simulink model "Final_Model_Building_2_AirflowAdded"  (R2022a)
settings: Solver=ode1  StartTime=0.0  StopTime=24*3600  FixedStep=10  RelTol=1e-3
values from neighbouring files (symbols this model uses):
  Aux_Threshold = 52    [Setup_Code_EWASP_VC.m]
  buildingAge = 2005    [Setup_Code_EWASP_VC.m]
  ceilingHeight = 2.4    [Setup_Code_EWASP_VC.m]
  conductiveHconnectMatrix = [ ... (first row only)    [Setup_Code_EWASP_VC.m]
  cRoofGreen = 100000    [Setup_Code_EWASP_VC.m]
  Defrost_After_Time = 30    [Setup_Code_EWASP_VC.m]
  DHWDemandProfile = occFreegainHotwaterElecTestPassiveOcc3(:,3)    [Setup_Code_EWASP_VC.m]
  Elec_Max = Elec_Max*(30/24.2)    [Setup_Code_EWASP_VC.m]
  Elec_Mid = Elec_Mid*(30/24.2)    [Setup_Code_EWASP_VC.m]
  Elec_Min = Elec_Min*(30/24.2)    [Setup_Code_EWASP_VC.m]
  ElecDemandProfile = occFreegainHotwaterElecTestPassiveOcc3(:,4)    [Setup_Code_EWASP_VC.m]
  ElecFixed = [Elec_Max(6,2) Elec_Max(6,4) Elec_Max(6,6) Elec_Max(6,7) ... (first row only)    [Setup_Code_EWASP_VC.m]
  floorOrCeilingArea = floorOrCeilingArea*1.15    [Setup_Code_EWASP_VC.m]
  forceCold = 0    [Setup_Code_EWASP_VC.m]
  freegain = occFreegainHotwaterElecTestPassiveOcc3(:,2)-max(occupancy)*25    [Setup_Code_EWASP_VC.m]
  furnitureModelOn = 1    [Setup_Code_EWASP_VC.m]
  Heat_Max = Heat_Max*(30/24.2)    [Setup_Code_EWASP_VC.m]
  Heat_Mid = Heat_Mid*(30/24.2)    [Setup_Code_EWASP_VC.m]
  Heat_Min = Heat_Min*(30/24.2)    [Setup_Code_EWASP_VC.m]
  HeatFixed = [Heat_Max(6,2) Heat_Max(6,4) Heat_Max(6,6) Heat_Max(6,7) ... (first row only)    [Setup_Code_EWASP_VC.m]
  HeatingOnProfile = repmat(HeatingOnProfile,365,1)    [Setup_Code_EWASP_VC.m]
  HEX_ReturnLowerLimit = 52.5    [Setup_Code_EWASP_VC.m]
  HEX_ReturnUpperLimit = 55    [Setup_Code_EWASP_VC.m]
  LeakMultiplier = 1+(2*(rand()-0.5)/10)    [Setup_Code_EWASP_VC.m]
  maxOcc = max(occupancyProfile)    [Setup_Code_EWASP_VC.m]
  NESW_wallArea = max(NESW_Lengths*ceilingHeight-NESW_Windows,0)    [Setup_Code_EWASP_VC.m]
  NESW_Windows = [ ... (first row only)    [Setup_Code_EWASP_VC.m]
  numRooms = roomCount    [Setup_Code_EWASP_VC.m]
  occupancy = occupancyProfile    [Setup_Code_EWASP_VC.m]
  offsetDays = 0    [Setup_Code_EWASP_VC.m]
  pumpChoice = pumpChoices(MinIndex,1)    [Setup_Code_EWASP_VC.m]
  pumpRamp = 180    [Setup_Code_EWASP_VC.m]
  ReturnLowerLimit = 37.5    [Setup_Code_EWASP_VC.m]
  ReturnUpperLimit = 40    [Setup_Code_EWASP_VC.m]
  RoofIrradiance = Flat_NS_EW_RoofIrradiance(:,1)    [Setup_Code_EWASP_VC.m]
  roofStartTemp = ones(11,1)*20    [Setup_Code_EWASP_VC.m]
  rooftype = 0    [Setup_Code_EWASP_VC.m]
  RoomDataMatrix = [zeros(1,12);ones(1,12)*wallDensity;zeros(1,12);ones(1,12)*wallU;ones(1,12)*windowU;ones(1,12)*floorU;ones(1,12)*ceilingU;zeros(1,12);windowArea, 0;floorOrCeilingArea;zeros(1,12);floorOrCeilingArea*ceilingHeight]    [Setup_Code_EWASP_VC.m]
  roomVol = roomVol*1.15    [Setup_Code_EWASP_VC.m]
  slabStartTemp = (GroundTempTimeSeries(offsetDays*1440+1,1)+thermostatSetting)/2    [Setup_Code_EWASP_VC.m]
  SlackRequest = zeros(1440,1)    [Setup_Code_EWASP_VC.m]
  SolarThermalExists = 0    [Setup_Code_EWASP_VC.m]
  SourceFixed = HeatFixed-ElecFixed    [Setup_Code_EWASP_VC.m]
  StateSeries = StateSeriesGenerator(22,7,1)    [Setup_Code_EWASP_VC.m]
  Tank_Lower_Temp = 49.5    [Setup_Code_EWASP_VC.m]
  Tank_Upper_Temp = 52    [Setup_Code_EWASP_VC.m]
  Tank_Volume_m3 = 0.15    [Setup_Code_EWASP_VC.m]
  TankHeatHour = randi([1 5])-1    [Setup_Code_EWASP_VC.m]
  upDown = [0;0;0;0;1;1;1;1;1;1;1]    [Setup_Code_EWASP_VC.m]
  wallStartTempExt = thermostatSetting*(0.266+0.00215*outdoorStartTemp+0.018*wallU+0.00113*outdoorStartTemp*wallU+0.0068*wallU^2)    [Setup_Code_EWASP_VC.m]
undefined symbols (not defined in the file or in its folder): a, ceilingU, condUDMatrix, convUDMatrix, deltaPEXPANDED_E, deltaPEXPANDED_E2, deltaPEXPANDED_N, deltaPEXPANDED_N2, deltaPEXPANDED_S, deltaPEXPANDED_S2, deltaPEXPANDED_W, deltaPEXPANDED_W2, DesiredDHWTemp, DesiredFlowTempVsInOutDeltaTemp, DiffuseHorizontal, DiscIntNeverNeededParam, DNI, dwnAndConcrete, DWORK_A_HX, DWORK_CHK_FLU, DWORK_CP_NODE, DWORK_DH, DWORK_FLUID, DWORK_HCON, DWORK_LOSS, DWORK_MDOTDOWN, DWORK_MDOTIN, DWORK_MDOTUP, DWORK_MIX, DWORK_PRESS, DWORK_QDOTIN, DWORK_RHO_NODE, DWORK_TIN, DWORK_TS_OLD, DWORK_V_NODE, ExtractRates, GroundTempTimeSeries, HCM, HCM2, HCM_closed, HCM_closed2, intermediateU, IsTop, massFlowMatrix, mechEfficiency, neighbourMatrix, numericalRoomUse, RadiatorMatrix, room2roomflowmatrix_E, room2roomflowmatrix_E2, room2roomflowmatrix_N, room2roomflowmatrix_N2, room2roomflowmatrix_S, room2roomflowmatrix_S2, room2roomflowmatrix_W, room2roomflowmatrix_W2, StateAirInEXPANDED_E, StateAirInEXPANDED_E2, StateAirInEXPANDED_N, StateAirInEXPANDED_N2 ... (+27)
libraries: simulink x6, dspsigops x4, dspmtrx3 x4, carnot x3, spsEdgeDetectorLib x2, dspstat3 x2, powerlib_meascontrol x1, simulink_extras x1
(part 21 of 27)

== system Final_Model_Building_2_AirflowAdded/Subsystem_Room3/Utility/Subsystem1/integrate deltat's with initial wall temps as initial condition ==
  In1 : Inport
  In2 : Inport  Port=2
  In3 : Inport  Port=3
  In4 : Inport  Port=4
  Constant : Constant  Value=2
  Constant1 : Constant
  Constant2 : Constant  Value=wallStartTempExt
  Discrete-Time Integrator : DiscreteIntegrator  InitialConditionSource=external  SampleTime=-1  ICPrevOutput=DiscIntNeverNeededParam  ICPrevScaledInput=DiscIntNeverNeededParam
  Discrete-Time Integrator1 : DiscreteIntegrator  InitialConditionSource=external  SampleTime=-1  ICPrevOutput=DiscIntNeverNeededParam  ICPrevScaledInput=DiscIntNeverNeededParam
  Discrete-Time Integrator2 : DiscreteIntegrator  InitialConditionSource=external  SampleTime=-1  ICPrevOutput=DiscIntNeverNeededParam  ICPrevScaledInput=DiscIntNeverNeededParam
  Display : Display
  Divide : Product  Inputs=*/
  Minus1 : Sum
  Minus2 : Sum  Inputs=+-
  Room Initial Temp Table : LookupNDDirect  NumberOfTableDimensions=1  Table=wallStartTempInt'
  Scope{,1..4} (5 alike) : Scope
  Out1 : Outport  VectorParamsAs1DForOutWhenUnconnected=off
  Out2 : Outport  Port=2  VectorParamsAs1DForOutWhenUnconnected=off
  Out3 : Outport  Port=3  VectorParamsAs1DForOutWhenUnconnected=off
  wires:
  Discrete-Time Integrator1/1 -> Scope1/1, Out2/1
  Discrete-Time Integrator2/1 -> Out1/1, Scope/1, Display/1
  Divide/1 -> Discrete-Time Integrator1/2
  In3/1 -> Discrete-Time Integrator/1
  Room Initial Temp Table/1 -> Discrete-Time Integrator2/2, Minus1/1, Scope3/1
  In2/1 -> Discrete-Time Integrator1/1
  Discrete-Time Integrator/1 -> Scope2/1, Out3/1
  Constant2/1 -> Discrete-Time Integrator/2, Minus1/2
  In1/1 -> Discrete-Time Integrator2/1
  In4/1 -> Scope4/1, Minus2/1
  Minus1/1 -> Divide/1
  Constant/1 -> Divide/2
  Constant1/1 -> Minus2/2
  Minus2/1 -> Room Initial Temp Table/1

== system Final_Model_Building_2_AirflowAdded/Subsystem_Room3/Utility/Subsystem3/integrate deltat's with initial wall temps as initial condition ==
  In1 : Inport
  In2 : Inport  Port=2
  In3 : Inport  Port=3
  In4 : Inport  Port=4
  Constant : Constant  Value=2
  Constant1 : Constant
  Constant2 : Constant  Value=wallStartTempExt
  Discrete-Time Integrator : DiscreteIntegrator  InitialConditionSource=external  SampleTime=-1  ICPrevOutput=DiscIntNeverNeededParam  ICPrevScaledInput=DiscIntNeverNeededParam
  Discrete-Time Integrator1 : DiscreteIntegrator  InitialConditionSource=external  SampleTime=-1  ICPrevOutput=DiscIntNeverNeededParam  ICPrevScaledInput=DiscIntNeverNeededParam
  Discrete-Time Integrator2 : DiscreteIntegrator  InitialConditionSource=external  SampleTime=-1  ICPrevOutput=DiscIntNeverNeededParam  ICPrevScaledInput=DiscIntNeverNeededParam
  Display : Display
  Divide : Product  Inputs=*/
  Minus1 : Sum
  Minus2 : Sum  Inputs=+-
  Room Initial Temp Table : LookupNDDirect  NumberOfTableDimensions=1  Table=roofStartTemp
  Scope{,1..2,4} (4 alike) : Scope
  Out1 : Outport  VectorParamsAs1DForOutWhenUnconnected=off
  Out2 : Outport  Port=2  VectorParamsAs1DForOutWhenUnconnected=off
  Out3 : Outport  Port=3  VectorParamsAs1DForOutWhenUnconnected=off
  wires:
  Discrete-Time Integrator1/1 -> Scope1/1, Out2/1
  Discrete-Time Integrator2/1 -> Out1/1, Scope/1, Display/1
  Divide/1 -> Discrete-Time Integrator1/2
  In3/1 -> Discrete-Time Integrator/1
  Room Initial Temp Table/1 -> Discrete-Time Integrator2/2, Minus1/1
  In2/1 -> Discrete-Time Integrator1/1
  Discrete-Time Integrator/1 -> Scope2/1, Out3/1
  Constant2/1 -> Discrete-Time Integrator/2, Minus1/2
  In1/1 -> Discrete-Time Integrator2/1
  In4/1 -> Scope4/1, Minus2/1
  Minus1/1 -> Divide/1
  Constant/1 -> Divide/2
  Constant1/1 -> Minus2/2
  Minus2/1 -> Room Initial Temp Table/1

== system Final_Model_Building_2_AirflowAdded/Subsystem_Room3/Utility/Subsystem4/Irradiance to Solar Gain1 ==
  note: Uses emperical relationship between incidence angle and irradiance through a double glazed window from: ' Simulating Thermochromic and Heat Mirror Glazing Systems in Hot and Cold Climates', G eorgios Kokogiannakis
      |
      | Uses equation for effective diffuse incidence angle from: 'Effective incidence angles of sky-diffuse and ground-reflected irradiance for various incidence angle modifier types', Ehud Strobach. the answer is then multiplied by the diffuse compontent of irradaiance, and also divided by (180-tilt) to account for the fact that only some of the diffuse irradiance is seen by the window (if tilted to 90 o then this is 0.5).
  In1 : Inport
  In2 : Inport  Port=2
  In3 : Inport  Port=3
  In4 : Inport  Port=4
  1-D Lookup Table : Lookup_n-D  NumberOfTableDimensions=1  BreakpointsForDimension1=[0,10,20,30,40,50,60,70,80,90]  Table=[0.53,0.525,0.52,0.51,0.495,0.47,0.415,0.31,0.14,0]  InternalRulePriority=Speed  RndMeth=Simplest
  1-D Lookup Table1 : Lookup_n-D  NumberOfTableDimensions=1  BreakpointsForDimension1=[0,10,20,30,40,50,60,70,80,90]  Table=[0.53,0.525,0.52,0.51,0.495,0.47,0.415,0.31,0.14,0]  InternalRulePriority=Speed  RndMeth=Simplest
  1-D Lookup Table2 : Lookup_n-D  NumberOfTableDimensions=1  BreakpointsForDimension1=[0,10,20,30,40,50,60,70,80,90]  Table=[0.04,0.04,0.04,0.04,0.05,0.05,0.08,0.175,0.38,1]  InternalRulePriority=Speed  RndMeth=Simplest
  1-D Lookup Table3 : Lookup_n-D  NumberOfTableDimensions=1  BreakpointsForDimension1=[0,10,20,30,40,50,60,70,80,90]  Table=[0.04,0.04,0.04,0.04,0.05,0.05,0.08,0.175,0.38,1]  InternalRulePriority=Speed  RndMeth=Simplest
  1-D Lookup Table4 : Lookup_n-D  NumberOfTableDimensions=1  BreakpointsForDimension1=[0,10,20,30,40,50,60,70,80,90]  Table=[0.43,0.435,0.44,0.45,0.455,0.48,0.505,0.515,0.48,0]  InternalRulePriority=Speed  RndMeth=Simplest
  1-D Lookup Table5 : Lookup_n-D  NumberOfTableDimensions=1  BreakpointsForDimension1=[0,10,20,30,40,50,60,70,80,90]  Table=[0.43,0.435,0.44,0.45,0.455,0.48,0.505,0.515,0.48,0]  InternalRulePriority=Speed  RndMeth=Simplest
  Add : Sum
  Add1 : Sum
  Add2 : Sum
  Constant : Constant  Value=180
  Constant1 : Constant  Value=180
  Constant2 : Constant  Value=180
  Fcn1 : Fcn  Expr=59.68-0.1457*u+0.001585*u^2
  Fcn2 : Fcn  Expr=59.68-0.1457*u+0.001585*u^2
  Fcn5 : Fcn  Expr=59.68-0.1457*u+0.001585*u^2
  Product1 : Product  Inputs=*/
  Product2 : Product
  Product3 : Product  Inputs=***
  Product4 : Product
  Product5 : Product  Inputs=*/
  Product6 : Product  Inputs=***
  Product7 : Product
  Product8 : Product  Inputs=***
  Product9 : Product  Inputs=*/
  Reflected portion not currently used : Terminator
  Sum : Sum  Inputs=|+-
  Sum1 : Sum  Inputs=|+-
  Sum2 : Sum  Inputs=|+-
  Out1 : Outport  VectorParamsAs1DForOutWhenUnconnected=off
  Out2 : Outport  Port=2  VectorParamsAs1DForOutWhenUnconnected=off
  wires:
  Product2/1 -> Add/1
  Fcn5/1 -> 1-D Lookup Table1/1
  Product3/1 -> Add/2
  In1/1 -> 1-D Lookup Table4/1, 1-D Lookup Table2/1, 1-D Lookup Table/1
  1-D Lookup Table1/1 -> Product3/1
  1-D Lookup Table/1 -> Product2/1
  Add/1 -> Out1/1
  Constant/1 -> Product1/2, Sum/1
  Sum/1 -> Product1/1
  Product1/1 -> Product3/3
  Product4/1 -> Add1/1
  1-D Lookup Table2/1 -> Product4/1
  In3/1 -> Product7/2, Product4/2, Product2/2
  Product5/1 -> Product6/3
  Constant1/1 -> Product5/2, Sum1/1
  1-D Lookup Table3/1 -> Product6/1
  Sum1/1 -> Product5/1
  Fcn1/1 -> 1-D Lookup Table3/1
  Product6/1 -> Add1/2
  Product7/1 -> Add2/1
  1-D Lookup Table4/1 -> Product7/1
  Product8/1 -> Add2/2
  Sum2/1 -> Product9/1
  Product9/1 -> Product8/3
  Constant2/1 -> Product9/2, Sum2/1
  In4/1 -> Product8/2, Product6/2, Product3/2
  1-D Lookup Table5/1 -> Product8/1
  Fcn2/1 -> 1-D Lookup Table5/1
  In2/1 -> Fcn1/1, Sum1/2, Fcn2/1, Sum2/2, Sum/2, Fcn5/1
  Add1/1 -> Reflected portion not currently used/1
  Add2/1 -> Out2/1

== system Final_Model_Building_2_AirflowAdded/Subsystem_Room4/Hall/Subsystem1/integrate deltat's with initial wall temps as initial condition ==
  In1 : Inport
  In2 : Inport  Port=2
  In3 : Inport  Port=3
  In4 : Inport  Port=4
  Constant : Constant  Value=2
  Constant1 : Constant
  Constant2 : Constant  Value=wallStartTempExt
  Discrete-Time Integrator : DiscreteIntegrator  InitialConditionSource=external  SampleTime=-1  ICPrevOutput=DiscIntNeverNeededParam  ICPrevScaledInput=DiscIntNeverNeededParam
  Discrete-Time Integrator1 : DiscreteIntegrator  InitialConditionSource=external  SampleTime=-1  ICPrevOutput=DiscIntNeverNeededParam  ICPrevScaledInput=DiscIntNeverNeededParam
  Discrete-Time Integrator2 : DiscreteIntegrator  InitialConditionSource=external  SampleTime=-1  ICPrevOutput=DiscIntNeverNeededParam  ICPrevScaledInput=DiscIntNeverNeededParam
  Display : Display
  Divide : Product  Inputs=*/
  Minus1 : Sum
  Minus2 : Sum  Inputs=+-
  Room Initial Temp Table : LookupNDDirect  NumberOfTableDimensions=1  Table=wallStartTempInt'
  Scope{,1..4} (5 alike) : Scope
  Out1 : Outport  VectorParamsAs1DForOutWhenUnconnected=off
  Out2 : Outport  Port=2  VectorParamsAs1DForOutWhenUnconnected=off
  Out3 : Outport  Port=3  VectorParamsAs1DForOutWhenUnconnected=off
  wires:
  Discrete-Time Integrator1/1 -> Scope1/1, Out2/1
  Discrete-Time Integrator2/1 -> Out1/1, Scope/1, Display/1
  Divide/1 -> Discrete-Time Integrator1/2
  In3/1 -> Discrete-Time Integrator/1
  Room Initial Temp Table/1 -> Discrete-Time Integrator2/2, Minus1/1, Scope3/1
  In2/1 -> Discrete-Time Integrator1/1
  Discrete-Time Integrator/1 -> Scope2/1, Out3/1
  Constant2/1 -> Discrete-Time Integrator/2, Minus1/2
  In1/1 -> Discrete-Time Integrator2/1
  In4/1 -> Scope4/1, Minus2/1
  Minus1/1 -> Divide/1
  Constant/1 -> Divide/2
  Constant1/1 -> Minus2/2
  Minus2/1 -> Room Initial Temp Table/1

== system Final_Model_Building_2_AirflowAdded/Subsystem_Room4/Hall/Subsystem3/integrate deltat's with initial wall temps as initial condition ==
  In1 : Inport
  In2 : Inport  Port=2
  In3 : Inport  Port=3
  In4 : Inport  Port=4
  Constant : Constant  Value=2
  Constant1 : Constant
  Constant2 : Constant  Value=wallStartTempExt
  Discrete-Time Integrator : DiscreteIntegrator  InitialConditionSource=external  SampleTime=-1  ICPrevOutput=DiscIntNeverNeededParam  ICPrevScaledInput=DiscIntNeverNeededParam
  Discrete-Time Integrator1 : DiscreteIntegrator  InitialConditionSource=external  SampleTime=-1  ICPrevOutput=DiscIntNeverNeededParam  ICPrevScaledInput=DiscIntNeverNeededParam
  Discrete-Time Integrator2 : DiscreteIntegrator  InitialConditionSource=external  SampleTime=-1  ICPrevOutput=DiscIntNeverNeededParam  ICPrevScaledInput=DiscIntNeverNeededParam
  Display : Display
  Divide : Product  Inputs=*/
  Minus1 : Sum
  Minus2 : Sum  Inputs=+-
  Room Initial Temp Table : LookupNDDirect  NumberOfTableDimensions=1  Table=roofStartTemp
  Scope{,1..2,4} (4 alike) : Scope
  Out1 : Outport  VectorParamsAs1DForOutWhenUnconnected=off
  Out2 : Outport  Port=2  VectorParamsAs1DForOutWhenUnconnected=off
  Out3 : Outport  Port=3  VectorParamsAs1DForOutWhenUnconnected=off
  wires:
  Discrete-Time Integrator1/1 -> Scope1/1, Out2/1
  Discrete-Time Integrator2/1 -> Out1/1, Scope/1, Display/1
  Divide/1 -> Discrete-Time Integrator1/2
  In3/1 -> Discrete-Time Integrator/1
  Room Initial Temp Table/1 -> Discrete-Time Integrator2/2, Minus1/1
  In2/1 -> Discrete-Time Integrator1/1
  Discrete-Time Integrator/1 -> Scope2/1, Out3/1
  Constant2/1 -> Discrete-Time Integrator/2, Minus1/2
  In1/1 -> Discrete-Time Integrator2/1
  In4/1 -> Scope4/1, Minus2/1
  Minus1/1 -> Divide/1
  Constant/1 -> Divide/2
  Constant1/1 -> Minus2/2
  Minus2/1 -> Room Initial Temp Table/1

== system Final_Model_Building_2_AirflowAdded/Subsystem_Room4/Hall/Subsystem4/Irradiance to Solar Gain1 ==
  note: Uses emperical relationship between incidence angle and irradiance through a double glazed window from: ' Simulating Thermochromic and Heat Mirror Glazing Systems in Hot and Cold Climates', G eorgios Kokogiannakis
      |
      | Uses equation for effective diffuse incidence angle from: 'Effective incidence angles of sky-diffuse and ground-reflected irradiance for various incidence angle modifier types', Ehud Strobach. the answer is then multiplied by the diffuse compontent of irradaiance, and also divided by (180-tilt) to account for the fact that only some of the diffuse irradiance is seen by the window (if tilted to 90 o then this is 0.5).
  In1 : Inport
  In2 : Inport  Port=2
  In3 : Inport  Port=3
  In4 : Inport  Port=4
  1-D Lookup Table : Lookup_n-D  NumberOfTableDimensions=1  BreakpointsForDimension1=[0,10,20,30,40,50,60,70,80,90]  Table=[0.53,0.525,0.52,0.51,0.495,0.47,0.415,0.31,0.14,0]  InternalRulePriority=Speed  RndMeth=Simplest
  1-D Lookup Table1 : Lookup_n-D  NumberOfTableDimensions=1  BreakpointsForDimension1=[0,10,20,30,40,50,60,70,80,90]  Table=[0.53,0.525,0.52,0.51,0.495,0.47,0.415,0.31,0.14,0]  InternalRulePriority=Speed  RndMeth=Simplest
  1-D Lookup Table2 : Lookup_n-D  NumberOfTableDimensions=1  BreakpointsForDimension1=[0,10,20,30,40,50,60,70,80,90]  Table=[0.04,0.04,0.04,0.04,0.05,0.05,0.08,0.175,0.38,1]  InternalRulePriority=Speed  RndMeth=Simplest
  1-D Lookup Table3 : Lookup_n-D  NumberOfTableDimensions=1  BreakpointsForDimension1=[0,10,20,30,40,50,60,70,80,90]  Table=[0.04,0.04,0.04,0.04,0.05,0.05,0.08,0.175,0.38,1]  InternalRulePriority=Speed  RndMeth=Simplest
  1-D Lookup Table4 : Lookup_n-D  NumberOfTableDimensions=1  BreakpointsForDimension1=[0,10,20,30,40,50,60,70,80,90]  Table=[0.43,0.435,0.44,0.45,0.455,0.48,0.505,0.515,0.48,0]  InternalRulePriority=Speed  RndMeth=Simplest
  1-D Lookup Table5 : Lookup_n-D  NumberOfTableDimensions=1  BreakpointsForDimension1=[0,10,20,30,40,50,60,70,80,90]  Table=[0.43,0.435,0.44,0.45,0.455,0.48,0.505,0.515,0.48,0]  InternalRulePriority=Speed  RndMeth=Simplest
  Add : Sum
  Add1 : Sum
  Add2 : Sum
  Constant : Constant  Value=180
  Constant1 : Constant  Value=180
  Constant2 : Constant  Value=180
  Fcn1 : Fcn  Expr=59.68-0.1457*u+0.001585*u^2
  Fcn2 : Fcn  Expr=59.68-0.1457*u+0.001585*u^2
  Fcn5 : Fcn  Expr=59.68-0.1457*u+0.001585*u^2
  Product1 : Product  Inputs=*/
  Product2 : Product
  Product3 : Product  Inputs=***
  Product4 : Product
  Product5 : Product  Inputs=*/
  Product6 : Product  Inputs=***
  Product7 : Product
  Product8 : Product  Inputs=***
  Product9 : Product  Inputs=*/
  Reflected portion not currently used : Terminator
  Sum : Sum  Inputs=|+-
  Sum1 : Sum  Inputs=|+-
  Sum2 : Sum  Inputs=|+-
  Out1 : Outport  VectorParamsAs1DForOutWhenUnconnected=off
  Out2 : Outport  Port=2  VectorParamsAs1DForOutWhenUnconnected=off
  wires:
  Product2/1 -> Add/1
  Fcn5/1 -> 1-D Lookup Table1/1
  Product3/1 -> Add/2
  In1/1 -> 1-D Lookup Table4/1, 1-D Lookup Table2/1, 1-D Lookup Table/1
  1-D Lookup Table1/1 -> Product3/1
  1-D Lookup Table/1 -> Product2/1
  Add/1 -> Out1/1
  Constant/1 -> Product1/2, Sum/1
  Sum/1 -> Product1/1
  Product1/1 -> Product3/3
  Product4/1 -> Add1/1
  1-D Lookup Table2/1 -> Product4/1
  In3/1 -> Product7/2, Product4/2, Product2/2
  Product5/1 -> Product6/3
  Constant1/1 -> Product5/2, Sum1/1
  1-D Lookup Table3/1 -> Product6/1
  Sum1/1 -> Product5/1
  Fcn1/1 -> 1-D Lookup Table3/1
  Product6/1 -> Add1/2
  Product7/1 -> Add2/1
  1-D Lookup Table4/1 -> Product7/1
  Product8/1 -> Add2/2
  Sum2/1 -> Product9/1
  Product9/1 -> Product8/3
  Constant2/1 -> Product9/2, Sum2/1
  In4/1 -> Product8/2, Product6/2, Product3/2
  1-D Lookup Table5/1 -> Product8/1
  Fcn2/1 -> 1-D Lookup Table5/1
  In2/1 -> Fcn1/1, Sum1/2, Fcn2/1, Sum2/2, Sum/2, Fcn5/1
  Add1/1 -> Reflected portion not currently used/1
  Add2/1 -> Out2/1

== system Final_Model_Building_2_AirflowAdded/Subsystem_Room5/Landing/Subsystem1/Irradiance to Solar Gain1 ==
  note: Uses emperical relationship between incidence angle and irradiance through a double glazed window from: ' Simulating Thermochromic and Heat Mirror Glazing Systems in Hot and Cold Climates', G eorgios Kokogiannakis
      |
      | Uses equation for effective diffuse incidence angle from: 'Effective incidence angles of sky-diffuse and ground-reflected irradiance for various incidence angle modifier types', Ehud Strobach. the answer is then multiplied by the diffuse compontent of irradaiance, and also divided by (180-tilt) to account for the fact that only some of the diffuse irradiance is seen by the window (if tilted to 90 o then this is 0.5).
  In1 : Inport
  In2 : Inport  Port=2
  In3 : Inport  Port=3
  In4 : Inport  Port=4
  1-D Lookup Table : Lookup_n-D  NumberOfTableDimensions=1  BreakpointsForDimension1=[0,10,20,30,40,50,60,70,80,90]  Table=[0.53,0.525,0.52,0.51,0.495,0.47,0.415,0.31,0.14,0]  InternalRulePriority=Speed  RndMeth=Simplest
  1-D Lookup Table1 : Lookup_n-D  NumberOfTableDimensions=1  BreakpointsForDimension1=[0,10,20,30,40,50,60,70,80,90]  Table=[0.53,0.525,0.52,0.51,0.495,0.47,0.415,0.31,0.14,0]  InternalRulePriority=Speed  RndMeth=Simplest
  1-D Lookup Table2 : Lookup_n-D  NumberOfTableDimensions=1  BreakpointsForDimension1=[0,10,20,30,40,50,60,70,80,90]  Table=[0.04,0.04,0.04,0.04,0.05,0.05,0.08,0.175,0.38,1]  InternalRulePriority=Speed  RndMeth=Simplest
  1-D Lookup Table3 : Lookup_n-D  NumberOfTableDimensions=1  BreakpointsForDimension1=[0,10,20,30,40,50,60,70,80,90]  Table=[0.04,0.04,0.04,0.04,0.05,0.05,0.08,0.175,0.38,1]  InternalRulePriority=Speed  RndMeth=Simplest
  1-D Lookup Table4 : Lookup_n-D  NumberOfTableDimensions=1  BreakpointsForDimension1=[0,10,20,30,40,50,60,70,80,90]  Table=[0.43,0.435,0.44,0.45,0.455,0.48,0.505,0.515,0.48,0]  InternalRulePriority=Speed  RndMeth=Simplest
  1-D Lookup Table5 : Lookup_n-D  NumberOfTableDimensions=1  BreakpointsForDimension1=[0,10,20,30,40,50,60,70,80,90]  Table=[0.43,0.435,0.44,0.45,0.455,0.48,0.505,0.515,0.48,0]  InternalRulePriority=Speed  RndMeth=Simplest
  Add : Sum
  Add1 : Sum
  Add2 : Sum
  Constant : Constant  Value=180
  Constant1 : Constant  Value=180
  Constant2 : Constant  Value=180
  Fcn1 : Fcn  Expr=59.68-0.1457*u+0.001585*u^2
  Fcn2 : Fcn  Expr=59.68-0.1457*u+0.001585*u^2
  Fcn5 : Fcn  Expr=59.68-0.1457*u+0.001585*u^2
  Product1 : Product  Inputs=*/
  Product2 : Product
  Product3 : Product  Inputs=***
  Product4 : Product
  Product5 : Product  Inputs=*/
  Product6 : Product  Inputs=***
  Product7 : Product
  Product8 : Product  Inputs=***
  Product9 : Product  Inputs=*/
  Reflected portion not currently used : Terminator
  Sum : Sum  Inputs=|+-
  Sum1 : Sum  Inputs=|+-
  Sum2 : Sum  Inputs=|+-
  Out1 : Outport  VectorParamsAs1DForOutWhenUnconnected=off
  Out2 : Outport  Port=2  VectorParamsAs1DForOutWhenUnconnected=off
  wires:
  Product2/1 -> Add/1
  Fcn5/1 -> 1-D Lookup Table1/1
  Product3/1 -> Add/2
  In1/1 -> 1-D Lookup Table4/1, 1-D Lookup Table2/1, 1-D Lookup Table/1
  1-D Lookup Table1/1 -> Product3/1
  1-D Lookup Table/1 -> Product2/1
  Add/1 -> Out1/1
  Constant/1 -> Product1/2, Sum/1
  Sum/1 -> Product1/1
  Product1/1 -> Product3/3
  Product4/1 -> Add1/1
  1-D Lookup Table2/1 -> Product4/1
  In3/1 -> Product7/2, Product4/2, Product2/2
  Product5/1 -> Product6/3
  Constant1/1 -> Product5/2, Sum1/1
  1-D Lookup Table3/1 -> Product6/1
  Sum1/1 -> Product5/1
  Fcn1/1 -> 1-D Lookup Table3/1
  Product6/1 -> Add1/2
  Product7/1 -> Add2/1
  1-D Lookup Table4/1 -> Product7/1
  Product8/1 -> Add2/2
  Sum2/1 -> Product9/1
  Product9/1 -> Product8/3
  Constant2/1 -> Product9/2, Sum2/1
  In4/1 -> Product8/2, Product6/2, Product3/2
  1-D Lookup Table5/1 -> Product8/1
  Fcn2/1 -> 1-D Lookup Table5/1
  In2/1 -> Fcn1/1, Sum1/2, Fcn2/1, Sum2/2, Sum/2, Fcn5/1
  Add1/1 -> Reflected portion not currently used/1
  Add2/1 -> Out2/1

== system Final_Model_Building_2_AirflowAdded/Subsystem_Room5/Landing/Subsystem2/integrate deltat's with initial wall temps as initial condition ==
  In1 : Inport
  In2 : Inport  Port=2
  In3 : Inport  Port=3
  In4 : Inport  Port=4
  Constant : Constant  Value=2
  Constant1 : Constant
  Constant2 : Constant  Value=wallStartTempExt
  Discrete-Time Integrator : DiscreteIntegrator  InitialConditionSource=external  SampleTime=-1  ICPrevOutput=DiscIntNeverNeededParam  ICPrevScaledInput=DiscIntNeverNeededParam
  Discrete-Time Integrator1 : DiscreteIntegrator  InitialConditionSource=external  SampleTime=-1  ICPrevOutput=DiscIntNeverNeededParam  ICPrevScaledInput=DiscIntNeverNeededParam
  Discrete-Time Integrator2 : DiscreteIntegrator  InitialConditionSource=external  SampleTime=-1  ICPrevOutput=DiscIntNeverNeededParam  ICPrevScaledInput=DiscIntNeverNeededParam
  Display : Display
  Divide : Product  Inputs=*/
  Minus1 : Sum
  Minus2 : Sum  Inputs=+-
  Room Initial Temp Table : LookupNDDirect  NumberOfTableDimensions=1  Table=wallStartTempInt'
  Scope{,1..4} (5 alike) : Scope
  Out1 : Outport  VectorParamsAs1DForOutWhenUnconnected=off
  Out2 : Outport  Port=2  VectorParamsAs1DForOutWhenUnconnected=off
  Out3 : Outport  Port=3  VectorParamsAs1DForOutWhenUnconnected=off
  wires:
  Discrete-Time Integrator1/1 -> Scope1/1, Out2/1
  Discrete-Time Integrator2/1 -> Out1/1, Scope/1, Display/1
  Divide/1 -> Discrete-Time Integrator1/2
  In3/1 -> Discrete-Time Integrator/1
  Room Initial Temp Table/1 -> Discrete-Time Integrator2/2, Minus1/1, Scope3/1
  In2/1 -> Discrete-Time Integrator1/1
  Discrete-Time Integrator/1 -> Scope2/1, Out3/1
  Constant2/1 -> Discrete-Time Integrator/2, Minus1/2
  In1/1 -> Discrete-Time Integrator2/1
  In4/1 -> Scope4/1, Minus2/1
  Minus1/1 -> Divide/1
  Constant/1 -> Divide/2
  Constant1/1 -> Minus2/2
  Minus2/1 -> Room Initial Temp Table/1

== system Final_Model_Building_2_AirflowAdded/Subsystem_Room5/Landing/Subsystem3/integrate deltat's with initial wall temps as initial condition ==
  In1 : Inport
  In2 : Inport  Port=2
  In3 : Inport  Port=3
  In4 : Inport  Port=4
  Constant : Constant  Value=2
  Constant1 : Constant
  Constant2 : Constant  Value=wallStartTempExt
  Discrete-Time Integrator : DiscreteIntegrator  InitialConditionSource=external  SampleTime=-1  ICPrevOutput=DiscIntNeverNeededParam  ICPrevScaledInput=DiscIntNeverNeededParam
  Discrete-Time Integrator1 : DiscreteIntegrator  InitialConditionSource=external  SampleTime=-1  ICPrevOutput=DiscIntNeverNeededParam  ICPrevScaledInput=DiscIntNeverNeededParam
  Discrete-Time Integrator2 : DiscreteIntegrator  InitialConditionSource=external  SampleTime=-1  ICPrevOutput=DiscIntNeverNeededParam  ICPrevScaledInput=DiscIntNeverNeededParam
  Display : Display
  Divide : Product  Inputs=*/
  Minus1 : Sum
  Minus2 : Sum  Inputs=+-
  Room Initial Temp Table : LookupNDDirect  NumberOfTableDimensions=1  Table=roofStartTemp
  Scope{,1..2,4} (4 alike) : Scope
  Out1 : Outport  VectorParamsAs1DForOutWhenUnconnected=off
  Out2 : Outport  Port=2  VectorParamsAs1DForOutWhenUnconnected=off
  Out3 : Outport  Port=3  VectorParamsAs1DForOutWhenUnconnected=off
  wires:
  Discrete-Time Integrator1/1 -> Scope1/1, Out2/1
  Discrete-Time Integrator2/1 -> Out1/1, Scope/1, Display/1
  Divide/1 -> Discrete-Time Integrator1/2
  In3/1 -> Discrete-Time Integrator/1
  Room Initial Temp Table/1 -> Discrete-Time Integrator2/2, Minus1/1
  In2/1 -> Discrete-Time Integrator1/1
  Discrete-Time Integrator/1 -> Scope2/1, Out3/1
  Constant2/1 -> Discrete-Time Integrator/2, Minus1/2
  In1/1 -> Discrete-Time Integrator2/1
  In4/1 -> Scope4/1, Minus2/1
  Minus1/1 -> Divide/1
  Constant/1 -> Divide/2
  Constant1/1 -> Minus2/2
  Minus2/1 -> Room Initial Temp Table/1

== system Final_Model_Building_2_AirflowAdded/Subsystem_Room6/Bedroom1/Subsystem1/integrate deltat's with initial wall temps as initial condition ==
  In1 : Inport
  In2 : Inport  Port=2
  In3 : Inport  Port=3
  In4 : Inport  Port=4
  Constant : Constant  Value=2
  Constant1 : Constant
  Constant2 : Constant  Value=wallStartTempExt
  Discrete-Time Integrator : DiscreteIntegrator  InitialConditionSource=external  SampleTime=-1  ICPrevOutput=DiscIntNeverNeededParam  ICPrevScaledInput=DiscIntNeverNeededParam
  Discrete-Time Integrator1 : DiscreteIntegrator  InitialConditionSource=external  SampleTime=-1  ICPrevOutput=DiscIntNeverNeededParam  ICPrevScaledInput=DiscIntNeverNeededParam
  Discrete-Time Integrator2 : DiscreteIntegrator  InitialConditionSource=external  SampleTime=-1  ICPrevOutput=DiscIntNeverNeededParam  ICPrevScaledInput=DiscIntNeverNeededParam
  Display : Display
  Divide : Product  Inputs=*/
  Minus1 : Sum
  Minus2 : Sum  Inputs=+-
  Room Initial Temp Table : LookupNDDirect  NumberOfTableDimensions=1  Table=wallStartTempInt'
  Scope{,1..4} (5 alike) : Scope
  Out1 : Outport  VectorParamsAs1DForOutWhenUnconnected=off
  Out2 : Outport  Port=2  VectorParamsAs1DForOutWhenUnconnected=off
  Out3 : Outport  Port=3  VectorParamsAs1DForOutWhenUnconnected=off
  wires:
  Discrete-Time Integrator1/1 -> Scope1/1, Out2/1
  Discrete-Time Integrator2/1 -> Out1/1, Scope/1, Display/1
  Divide/1 -> Discrete-Time Integrator1/2
  In3/1 -> Discrete-Time Integrator/1
  Room Initial Temp Table/1 -> Discrete-Time Integrator2/2, Minus1/1, Scope3/1
  In2/1 -> Discrete-Time Integrator1/1
  Discrete-Time Integrator/1 -> Scope2/1, Out3/1
  Constant2/1 -> Discrete-Time Integrator/2, Minus1/2
  In1/1 -> Discrete-Time Integrator2/1
  In4/1 -> Scope4/1, Minus2/1
  Minus1/1 -> Divide/1
  Constant/1 -> Divide/2
  Constant1/1 -> Minus2/2
  Minus2/1 -> Room Initial Temp Table/1

== system Final_Model_Building_2_AirflowAdded/Subsystem_Room6/Bedroom1/Subsystem2/Irradiance to Solar Gain1 ==
  note: Uses emperical relationship between incidence angle and irradiance through a double glazed window from: ' Simulating Thermochromic and Heat Mirror Glazing Systems in Hot and Cold Climates', G eorgios Kokogiannakis
      |
      | Uses equation for effective diffuse incidence angle from: 'Effective incidence angles of sky-diffuse and ground-reflected irradiance for various incidence angle modifier types', Ehud Strobach. the answer is then multiplied by the diffuse compontent of irradaiance, and also divided by (180-tilt) to account for the fact that only some of the diffuse irradiance is seen by the window (if tilted to 90 o then this is 0.5).
  In1 : Inport
  In2 : Inport  Port=2
  In3 : Inport  Port=3
  In4 : Inport  Port=4
  1-D Lookup Table : Lookup_n-D  NumberOfTableDimensions=1  BreakpointsForDimension1=[0,10,20,30,40,50,60,70,80,90]  Table=[0.53,0.525,0.52,0.51,0.495,0.47,0.415,0.31,0.14,0]  InternalRulePriority=Speed  RndMeth=Simplest
  1-D Lookup Table1 : Lookup_n-D  NumberOfTableDimensions=1  BreakpointsForDimension1=[0,10,20,30,40,50,60,70,80,90]  Table=[0.53,0.525,0.52,0.51,0.495,0.47,0.415,0.31,0.14,0]  InternalRulePriority=Speed  RndMeth=Simplest
  1-D Lookup Table2 : Lookup_n-D  NumberOfTableDimensions=1  BreakpointsForDimension1=[0,10,20,30,40,50,60,70,80,90]  Table=[0.04,0.04,0.04,0.04,0.05,0.05,0.08,0.175,0.38,1]  InternalRulePriority=Speed  RndMeth=Simplest
  1-D Lookup Table3 : Lookup_n-D  NumberOfTableDimensions=1  BreakpointsForDimension1=[0,10,20,30,40,50,60,70,80,90]  Table=[0.04,0.04,0.04,0.04,0.05,0.05,0.08,0.175,0.38,1]  InternalRulePriority=Speed  RndMeth=Simplest
  1-D Lookup Table4 : Lookup_n-D  NumberOfTableDimensions=1  BreakpointsForDimension1=[0,10,20,30,40,50,60,70,80,90]  Table=[0.43,0.435,0.44,0.45,0.455,0.48,0.505,0.515,0.48,0]  InternalRulePriority=Speed  RndMeth=Simplest
  1-D Lookup Table5 : Lookup_n-D  NumberOfTableDimensions=1  BreakpointsForDimension1=[0,10,20,30,40,50,60,70,80,90]  Table=[0.43,0.435,0.44,0.45,0.455,0.48,0.505,0.515,0.48,0]  InternalRulePriority=Speed  RndMeth=Simplest
  Add : Sum
  Add1 : Sum
  Add2 : Sum
  Constant : Constant  Value=180
  Constant1 : Constant  Value=180
  Constant2 : Constant  Value=180
  Fcn1 : Fcn  Expr=59.68-0.1457*u+0.001585*u^2
  Fcn2 : Fcn  Expr=59.68-0.1457*u+0.001585*u^2
  Fcn5 : Fcn  Expr=59.68-0.1457*u+0.001585*u^2
  Product1 : Product  Inputs=*/
  Product2 : Product
  Product3 : Product  Inputs=***
  Product4 : Product
  Product5 : Product  Inputs=*/
  Product6 : Product  Inputs=***
  Product7 : Product
  Product8 : Product  Inputs=***
  Product9 : Product  Inputs=*/
  Reflected portion not currently used : Terminator
  Sum : Sum  Inputs=|+-
  Sum1 : Sum  Inputs=|+-
  Sum2 : Sum  Inputs=|+-
  Out1 : Outport  VectorParamsAs1DForOutWhenUnconnected=off
  Out2 : Outport  Port=2  VectorParamsAs1DForOutWhenUnconnected=off
  wires:
  Product2/1 -> Add/1
  Fcn5/1 -> 1-D Lookup Table1/1
  Product3/1 -> Add/2
  In1/1 -> 1-D Lookup Table4/1, 1-D Lookup Table2/1, 1-D Lookup Table/1
  1-D Lookup Table1/1 -> Product3/1
  1-D Lookup Table/1 -> Product2/1
  Add/1 -> Out1/1
  Constant/1 -> Product1/2, Sum/1
  Sum/1 -> Product1/1
  Product1/1 -> Product3/3
  Product4/1 -> Add1/1
  1-D Lookup Table2/1 -> Product4/1
  In3/1 -> Product7/2, Product4/2, Product2/2
  Product5/1 -> Product6/3
  Constant1/1 -> Product5/2, Sum1/1
  1-D Lookup Table3/1 -> Product6/1
  Sum1/1 -> Product5/1
  Fcn1/1 -> 1-D Lookup Table3/1
  Product6/1 -> Add1/2
  Product7/1 -> Add2/1
  1-D Lookup Table4/1 -> Product7/1
  Product8/1 -> Add2/2
  Sum2/1 -> Product9/1
  Product9/1 -> Product8/3
  Constant2/1 -> Product9/2, Sum2/1
  In4/1 -> Product8/2, Product6/2, Product3/2
  1-D Lookup Table5/1 -> Product8/1
  Fcn2/1 -> 1-D Lookup Table5/1
  In2/1 -> Fcn1/1, Sum1/2, Fcn2/1, Sum2/2, Sum/2, Fcn5/1
  Add1/1 -> Reflected portion not currently used/1
  Add2/1 -> Out2/1

== system Final_Model_Building_2_AirflowAdded/Subsystem_Room6/Bedroom1/Subsystem3/integrate deltat's with initial wall temps as initial condition ==
  In1 : Inport
  In2 : Inport  Port=2
  In3 : Inport  Port=3
  In4 : Inport  Port=4
  Constant : Constant  Value=2
  Constant1 : Constant
  Constant2 : Constant  Value=wallStartTempExt
  Discrete-Time Integrator : DiscreteIntegrator  InitialConditionSource=external  SampleTime=-1  ICPrevOutput=DiscIntNeverNeededParam  ICPrevScaledInput=DiscIntNeverNeededParam
  Discrete-Time Integrator1 : DiscreteIntegrator  InitialConditionSource=external  SampleTime=-1  ICPrevOutput=DiscIntNeverNeededParam  ICPrevScaledInput=DiscIntNeverNeededParam
  Discrete-Time Integrator2 : DiscreteIntegrator  InitialConditionSource=external  SampleTime=-1  ICPrevOutput=DiscIntNeverNeededParam  ICPrevScaledInput=DiscIntNeverNeededParam
  Display : Display
  Divide : Product  Inputs=*/
  Minus1 : Sum
  Minus2 : Sum  Inputs=+-
  Room Initial Temp Table : LookupNDDirect  NumberOfTableDimensions=1  Table=roofStartTemp
  Scope{,1..2,4} (4 alike) : Scope
  Out1 : Outport  VectorParamsAs1DForOutWhenUnconnected=off
  Out2 : Outport  Port=2  VectorParamsAs1DForOutWhenUnconnected=off
  Out3 : Outport  Port=3  VectorParamsAs1DForOutWhenUnconnected=off
  wires:
  Discrete-Time Integrator1/1 -> Scope1/1, Out2/1
  Discrete-Time Integrator2/1 -> Out1/1, Scope/1, Display/1
  Divide/1 -> Discrete-Time Integrator1/2
  In3/1 -> Discrete-Time Integrator/1
  Room Initial Temp Table/1 -> Discrete-Time Integrator2/2, Minus1/1
  In2/1 -> Discrete-Time Integrator1/1
  Discrete-Time Integrator/1 -> Scope2/1, Out3/1
  Constant2/1 -> Discrete-Time Integrator/2, Minus1/2
  In1/1 -> Discrete-Time Integrator2/1
  In4/1 -> Scope4/1, Minus2/1
  Minus1/1 -> Divide/1
  Constant/1 -> Divide/2
  Constant1/1 -> Minus2/2
  Minus2/1 -> Room Initial Temp Table/1

== system Final_Model_Building_2_AirflowAdded/Subsystem_Room7/Bedroom 2/Subsystem1/integrate deltat's with initial wall temps as initial condition ==
  In1 : Inport
  In2 : Inport  Port=2
  In3 : Inport  Port=3
  In4 : Inport  Port=4
  Constant : Constant  Value=2
  Constant1 : Constant
  Constant2 : Constant  Value=wallStartTempExt
  Discrete-Time Integrator : DiscreteIntegrator  InitialConditionSource=external  SampleTime=-1  ICPrevOutput=DiscIntNeverNeededParam  ICPrevScaledInput=DiscIntNeverNeededParam
  Discrete-Time Integrator1 : DiscreteIntegrator  InitialConditionSource=external  SampleTime=-1  ICPrevOutput=DiscIntNeverNeededParam  ICPrevScaledInput=DiscIntNeverNeededParam
  Discrete-Time Integrator2 : DiscreteIntegrator  InitialConditionSource=external  SampleTime=-1  ICPrevOutput=DiscIntNeverNeededParam  ICPrevScaledInput=DiscIntNeverNeededParam
  Display : Display
  Divide : Product  Inputs=*/
  Minus1 : Sum
  Minus2 : Sum  Inputs=+-
  Room Initial Temp Table : LookupNDDirect  NumberOfTableDimensions=1  Table=roofStartTemp
  Scope{,1..2,4} (4 alike) : Scope
  Out1 : Outport  VectorParamsAs1DForOutWhenUnconnected=off
  Out2 : Outport  Port=2  VectorParamsAs1DForOutWhenUnconnected=off
  Out3 : Outport  Port=3  VectorParamsAs1DForOutWhenUnconnected=off
  wires:
  Discrete-Time Integrator1/1 -> Scope1/1, Out2/1
  Discrete-Time Integrator2/1 -> Out1/1, Scope/1, Display/1
  Divide/1 -> Discrete-Time Integrator1/2
  In3/1 -> Discrete-Time Integrator/1
  Room Initial Temp Table/1 -> Discrete-Time Integrator2/2, Minus1/1
  In2/1 -> Discrete-Time Integrator1/1
  Discrete-Time Integrator/1 -> Scope2/1, Out3/1
  Constant2/1 -> Discrete-Time Integrator/2, Minus1/2
  In1/1 -> Discrete-Time Integrator2/1
  In4/1 -> Scope4/1, Minus2/1
  Minus1/1 -> Divide/1
  Constant/1 -> Divide/2
  Constant1/1 -> Minus2/2
  Minus2/1 -> Room Initial Temp Table/1

== system Final_Model_Building_2_AirflowAdded/Subsystem_Room7/Bedroom 2/Subsystem3/integrate deltat's with initial wall temps as initial condition ==
  In1 : Inport
  In2 : Inport  Port=2
  In3 : Inport  Port=3
  In4 : Inport  Port=4
  Constant : Constant  Value=2
  Constant1 : Constant
  Constant2 : Constant  Value=wallStartTempExt
  Discrete-Time Integrator : DiscreteIntegrator  InitialConditionSource=external  SampleTime=-1  ICPrevOutput=DiscIntNeverNeededParam  ICPrevScaledInput=DiscIntNeverNeededParam
  Discrete-Time Integrator1 : DiscreteIntegrator  InitialConditionSource=external  SampleTime=-1  ICPrevOutput=DiscIntNeverNeededParam  ICPrevScaledInput=DiscIntNeverNeededParam
  Discrete-Time Integrator2 : DiscreteIntegrator  InitialConditionSource=external  SampleTime=-1  ICPrevOutput=DiscIntNeverNeededParam  ICPrevScaledInput=DiscIntNeverNeededParam
  Display : Display
  Divide : Product  Inputs=*/
  Minus1 : Sum
  Minus2 : Sum  Inputs=+-
  Room Initial Temp Table : LookupNDDirect  NumberOfTableDimensions=1  Table=wallStartTempInt'
  Scope{,1..4} (5 alike) : Scope
  Out1 : Outport  VectorParamsAs1DForOutWhenUnconnected=off
  Out2 : Outport  Port=2  VectorParamsAs1DForOutWhenUnconnected=off
  Out3 : Outport  Port=3  VectorParamsAs1DForOutWhenUnconnected=off
  wires:
  Discrete-Time Integrator1/1 -> Scope1/1, Out2/1
  Discrete-Time Integrator2/1 -> Out1/1, Scope/1, Display/1
  Divide/1 -> Discrete-Time Integrator1/2
  In3/1 -> Discrete-Time Integrator/1
  Room Initial Temp Table/1 -> Discrete-Time Integrator2/2, Minus1/1, Scope3/1
  In2/1 -> Discrete-Time Integrator1/1
  Discrete-Time Integrator/1 -> Scope2/1, Out3/1
  Constant2/1 -> Discrete-Time Integrator/2, Minus1/2
  In1/1 -> Discrete-Time Integrator2/1
  In4/1 -> Scope4/1, Minus2/1
  Minus1/1 -> Divide/1
  Constant/1 -> Divide/2
  Constant1/1 -> Minus2/2
  Minus2/1 -> Room Initial Temp Table/1

== system Final_Model_Building_2_AirflowAdded/Subsystem_Room7/Bedroom 2/Subsystem4/Irradiance to Solar Gain1 ==
  note: Uses emperical relationship between incidence angle and irradiance through a double glazed window from: ' Simulating Thermochromic and Heat Mirror Glazing Systems in Hot and Cold Climates', G eorgios Kokogiannakis
      |
      | Uses equation for effective diffuse incidence angle from: 'Effective incidence angles of sky-diffuse and ground-reflected irradiance for various incidence angle modifier types', Ehud Strobach. the answer is then multiplied by the diffuse compontent of irradaiance, and also divided by (180-tilt) to account for the fact that only some of the diffuse irradiance is seen by the window (if tilted to 90 o then this is 0.5).
  In1 : Inport
  In2 : Inport  Port=2
  In3 : Inport  Port=3
  In4 : Inport  Port=4
  1-D Lookup Table : Lookup_n-D  NumberOfTableDimensions=1  BreakpointsForDimension1=[0,10,20,30,40,50,60,70,80,90]  Table=[0.53,0.525,0.52,0.51,0.495,0.47,0.415,0.31,0.14,0]  InternalRulePriority=Speed  RndMeth=Simplest
  1-D Lookup Table1 : Lookup_n-D  NumberOfTableDimensions=1  BreakpointsForDimension1=[0,10,20,30,40,50,60,70,80,90]  Table=[0.53,0.525,0.52,0.51,0.495,0.47,0.415,0.31,0.14,0]  InternalRulePriority=Speed  RndMeth=Simplest
  1-D Lookup Table2 : Lookup_n-D  NumberOfTableDimensions=1  BreakpointsForDimension1=[0,10,20,30,40,50,60,70,80,90]  Table=[0.04,0.04,0.04,0.04,0.05,0.05,0.08,0.175,0.38,1]  InternalRulePriority=Speed  RndMeth=Simplest
  1-D Lookup Table3 : Lookup_n-D  NumberOfTableDimensions=1  BreakpointsForDimension1=[0,10,20,30,40,50,60,70,80,90]  Table=[0.04,0.04,0.04,0.04,0.05,0.05,0.08,0.175,0.38,1]  InternalRulePriority=Speed  RndMeth=Simplest
  1-D Lookup Table4 : Lookup_n-D  NumberOfTableDimensions=1  BreakpointsForDimension1=[0,10,20,30,40,50,60,70,80,90]  Table=[0.43,0.435,0.44,0.45,0.455,0.48,0.505,0.515,0.48,0]  InternalRulePriority=Speed  RndMeth=Simplest
  1-D Lookup Table5 : Lookup_n-D  NumberOfTableDimensions=1  BreakpointsForDimension1=[0,10,20,30,40,50,60,70,80,90]  Table=[0.43,0.435,0.44,0.45,0.455,0.48,0.505,0.515,0.48,0]  InternalRulePriority=Speed  RndMeth=Simplest
  Add : Sum
  Add1 : Sum
  Add2 : Sum
  Constant : Constant  Value=180
  Constant1 : Constant  Value=180
  Constant2 : Constant  Value=180
  Fcn1 : Fcn  Expr=59.68-0.1457*u+0.001585*u^2
  Fcn2 : Fcn  Expr=59.68-0.1457*u+0.001585*u^2
  Fcn5 : Fcn  Expr=59.68-0.1457*u+0.001585*u^2
  Product1 : Product  Inputs=*/
  Product2 : Product
  Product3 : Product  Inputs=***
  Product4 : Product
  Product5 : Product  Inputs=*/
  Product6 : Product  Inputs=***
  Product7 : Product
  Product8 : Product  Inputs=***
  Product9 : Product  Inputs=*/
  Reflected portion not currently used : Terminator
  Sum : Sum  Inputs=|+-
  Sum1 : Sum  Inputs=|+-
  Sum2 : Sum  Inputs=|+-
  Out1 : Outport  VectorParamsAs1DForOutWhenUnconnected=off
  Out2 : Outport  Port=2  VectorParamsAs1DForOutWhenUnconnected=off
  wires:
  Product2/1 -> Add/1
  Fcn5/1 -> 1-D Lookup Table1/1
  Product3/1 -> Add/2
  In1/1 -> 1-D Lookup Table4/1, 1-D Lookup Table2/1, 1-D Lookup Table/1
  1-D Lookup Table1/1 -> Product3/1
  1-D Lookup Table/1 -> Product2/1
  Add/1 -> Out1/1
  Constant/1 -> Product1/2, Sum/1
  Sum/1 -> Product1/1
  Product1/1 -> Product3/3
  Product4/1 -> Add1/1
  1-D Lookup Table2/1 -> Product4/1
  In3/1 -> Product7/2, Product4/2, Product2/2
  Product5/1 -> Product6/3
  Constant1/1 -> Product5/2, Sum1/1
  1-D Lookup Table3/1 -> Product6/1
  Sum1/1 -> Product5/1
  Fcn1/1 -> 1-D Lookup Table3/1
  Product6/1 -> Add1/2
  Product7/1 -> Add2/1
  1-D Lookup Table4/1 -> Product7/1
  Product8/1 -> Add2/2
  Sum2/1 -> Product9/1
  Product9/1 -> Product8/3
  Constant2/1 -> Product9/2, Sum2/1
  In4/1 -> Product8/2, Product6/2, Product3/2
  1-D Lookup Table5/1 -> Product8/1
  Fcn2/1 -> 1-D Lookup Table5/1
  In2/1 -> Fcn1/1, Sum1/2, Fcn2/1, Sum2/2, Sum/2, Fcn5/1
  Add1/1 -> Reflected portion not currently used/1
  Add2/1 -> Out2/1

== system Final_Model_Building_2_AirflowAdded/Subsystem_Room8/Bedroom3/Subsystem1/integrate deltat's with initial wall temps as initial condition ==
  In1 : Inport
  In2 : Inport  Port=2
  In3 : Inport  Port=3
  In4 : Inport  Port=4
  Constant : Constant  Value=2
  Constant1 : Constant
  Constant2 : Constant  Value=wallStartTempExt
  Discrete-Time Integrator : DiscreteIntegrator  InitialConditionSource=external  SampleTime=-1  ICPrevOutput=DiscIntNeverNeededParam  ICPrevScaledInput=DiscIntNeverNeededParam
  Discrete-Time Integrator1 : DiscreteIntegrator  InitialConditionSource=external  SampleTime=-1  ICPrevOutput=DiscIntNeverNeededParam  ICPrevScaledInput=DiscIntNeverNeededParam
  Discrete-Time Integrator2 : DiscreteIntegrator  InitialConditionSource=external  SampleTime=-1  ICPrevOutput=DiscIntNeverNeededParam  ICPrevScaledInput=DiscIntNeverNeededParam
  Display : Display
  Divide : Product  Inputs=*/
  Minus1 : Sum
  Minus2 : Sum  Inputs=+-
  Room Initial Temp Table : LookupNDDirect  NumberOfTableDimensions=1  Table=wallStartTempInt'
  Scope{,1..4} (5 alike) : Scope
  Out1 : Outport  VectorParamsAs1DForOutWhenUnconnected=off
  Out2 : Outport  Port=2  VectorParamsAs1DForOutWhenUnconnected=off
  Out3 : Outport  Port=3  VectorParamsAs1DForOutWhenUnconnected=off
  wires:
  Discrete-Time Integrator1/1 -> Scope1/1, Out2/1
  Discrete-Time Integrator2/1 -> Out1/1, Scope/1, Display/1
  Divide/1 -> Discrete-Time Integrator1/2
  In3/1 -> Discrete-Time Integrator/1
  Room Initial Temp Table/1 -> Discrete-Time Integrator2/2, Minus1/1, Scope3/1
  In2/1 -> Discrete-Time Integrator1/1
  Discrete-Time Integrator/1 -> Scope2/1, Out3/1
  Constant2/1 -> Discrete-Time Integrator/2, Minus1/2
  In1/1 -> Discrete-Time Integrator2/1
  In4/1 -> Scope4/1, Minus2/1
  Minus1/1 -> Divide/1
  Constant/1 -> Divide/2
  Constant1/1 -> Minus2/2
  Minus2/1 -> Room Initial Temp Table/1

== system Final_Model_Building_2_AirflowAdded/Subsystem_Room8/Bedroom3/Subsystem3/integrate deltat's with initial wall temps as initial condition ==
  In1 : Inport
  In2 : Inport  Port=2
  In3 : Inport  Port=3
  In4 : Inport  Port=4
  Constant : Constant  Value=2
  Constant1 : Constant
  Constant2 : Constant  Value=wallStartTempExt
  Discrete-Time Integrator : DiscreteIntegrator  InitialConditionSource=external  SampleTime=-1  ICPrevOutput=DiscIntNeverNeededParam  ICPrevScaledInput=DiscIntNeverNeededParam
  Discrete-Time Integrator1 : DiscreteIntegrator  InitialConditionSource=external  SampleTime=-1  ICPrevOutput=DiscIntNeverNeededParam  ICPrevScaledInput=DiscIntNeverNeededParam
  Discrete-Time Integrator2 : DiscreteIntegrator  InitialConditionSource=external  SampleTime=-1  ICPrevOutput=DiscIntNeverNeededParam  ICPrevScaledInput=DiscIntNeverNeededParam
  Display : Display
  Divide : Product  Inputs=*/
  Minus1 : Sum
  Minus2 : Sum  Inputs=+-
  Room Initial Temp Table : LookupNDDirect  NumberOfTableDimensions=1  Table=roofStartTemp
  Scope{,1..2,4} (4 alike) : Scope
  Out1 : Outport  VectorParamsAs1DForOutWhenUnconnected=off
  Out2 : Outport  Port=2  VectorParamsAs1DForOutWhenUnconnected=off
  Out3 : Outport  Port=3  VectorParamsAs1DForOutWhenUnconnected=off
  wires:
  Discrete-Time Integrator1/1 -> Scope1/1, Out2/1
  Discrete-Time Integrator2/1 -> Out1/1, Scope/1, Display/1
  Divide/1 -> Discrete-Time Integrator1/2
  In3/1 -> Discrete-Time Integrator/1
  Room Initial Temp Table/1 -> Discrete-Time Integrator2/2, Minus1/1
  In2/1 -> Discrete-Time Integrator1/1
  Discrete-Time Integrator/1 -> Scope2/1, Out3/1
  Constant2/1 -> Discrete-Time Integrator/2, Minus1/2
  In1/1 -> Discrete-Time Integrator2/1
  In4/1 -> Scope4/1, Minus2/1
  Minus1/1 -> Divide/1
  Constant/1 -> Divide/2
  Constant1/1 -> Minus2/2
  Minus2/1 -> Room Initial Temp Table/1
